simulink model "Playground"  (R2021b)
settings: Solver=ode23t  StartTime=0.0  StopTime=inf  RelTol=1e-3
InitFcn:
  | RPInit
model workspace (MAT data in the model file):
  mapForSim : object (value not decoded)
  occGrid : robotics.BinaryOccupancyGrid (value not decoded)
undefined symbols (not defined in the file or in its folder): X, Y, Z
libraries: sm_lib x25, nesl_utility x11, RP_Simulator_Components x7, ME598_ProjectLibrary x6, RoboticsPlayground x2, Contact_Forces_Lib x2
(part 2 of 2)

== matlab function Playground/-180* : 180*1 ==
  data: deg input; deg output
function deg = degWrap(deg)

% % Convert radians to degrees
% deg = 180/pi * rad;


% Wrap degree value to the range -180* : +180*
for idx = 1:length(deg)
    while deg(idx) < -180
        deg(idx) = deg(idx)+360;
    end
    
    while deg(idx) > 180
        deg(idx) = deg(idx)-360;
    end
end

return

== matlab function Playground/MATLAB Function1 ==
  data: x input; y input; LeftM output; t input; RightM output; theta output
function [LeftM,RightM,theta] = fcn(x, y, t)
theta = atan2d((1.5-y),(0-x));
LeftM = -50;
RightM = 50;
while (t < theta+2 && t > theta-2)
    LeftM = 80;
    RightM = 80;
end

== matlab function Playground/MATLAB Function ==
  data: leftMotor output; rightMotor output; Left_Distance input; Front_Distance input; Right_Distance input
function [leftMotor, rightMotor] = test (Left_Distance, Front_Distance, Right_Distance)

    if (Front_Distance < 0.5)
        leftMotor = -100;
        rightMotor = 100;
    
    elseif (Front_Distance < 0.5 && Right_Distance < 0.5)
            leftMotor = -100;
            rightMotor = 100;

    elseif (Right_Distance < 0.5)
            leftMotor = -100;
            rightMotor = 100;
    else
        leftMotor = 100;
        rightMotor = 100;

    end
